simulink model "Test_21"  (R2024b)
settings: Solver=FixedStepAuto  StartTime=0.0  StopTime=50  RelTol=1e-3
undefined symbols (not defined in the file): BOOL, DINT, OTL, slplc
libraries: arduinolib x4
(part 2 of 10)

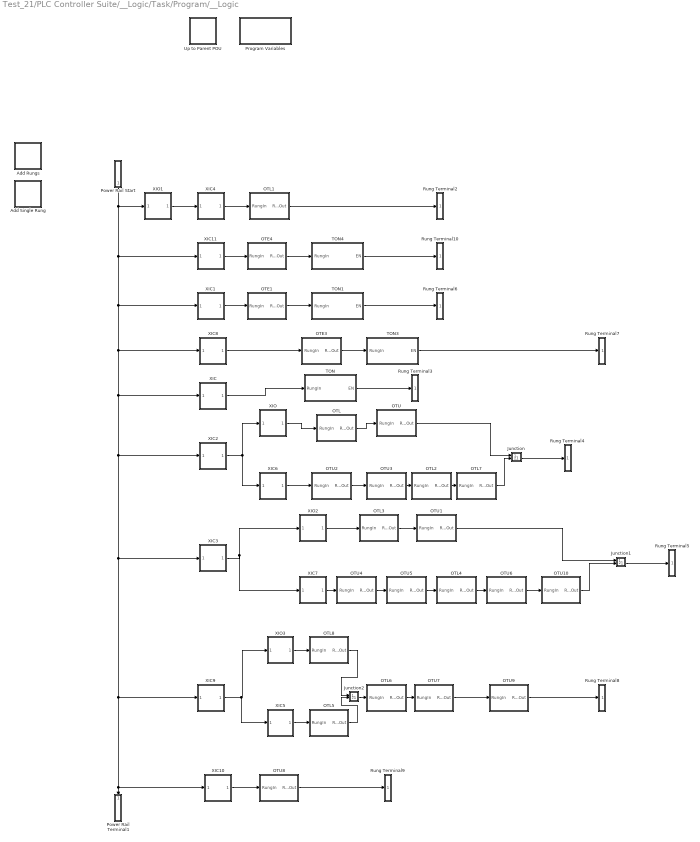
== system Test_21/PLC Controller Suite/__Logic/Task/Program/__Logic ==
  Add Rungs : Subsystem  DisableCoverage=on  TreatAsAtomicUnit=on  mask{PLCRungNumberToAdd=2, PLCBlockType=AddRungs}
      mask prompts: PLCRungNumberToAdd "Rung Number:"
      mask Help: web([docroot '/plccoder/ref/addrungs' '.html']);
      mask DialogControl PLCAddRungs Prompt: Add Rungs
      mask DialogControl PLCRungAddButton Prompt: Add
      mask DialogControl PLCRungAddButton Callback: slplc.callbacks.addLadderRungs(gcb);
      mask Display: disp(sprintf(['Add' newline 'Rungs']));
  Add Single Rung : Subsystem  DisableCoverage=on  TreatAsAtomicUnit=on  mask{PLCRungNumberToAdd=1, PLCBlockType=AddSingleRung}
      settings: OpenFcn=slplc.callbacks.addLadderRungs(gcb);
      mask Help: web([docroot '/plccoder/ref/addsinglerung' '.html']);
      mask DialogControl PLCAddRung Prompt: Add Single Rung
      mask Display: disp(sprintf(['Add' newline '1 Rung']));
  Junction : Subsystem  Priority=30  DisableCoverage=on  TreatAsAtomicUnit=on  mask{PLCBlockType=Junction, PLCPOUType=BranchJunction}
      mask Help: web([docroot '/plccoder/ref/junction' '.html']);
      mask DialogControl PLCBlockTitle Prompt: Rung Merge Point
      mask DialogControl PLCBlockDesc Prompt: This is the ladder diagram rung merge point.
  Junction1 : Subsystem  Priority=42  DisableCoverage=on  TreatAsAtomicUnit=on  mask{PLCBlockType=Junction, PLCPOUType=BranchJunction}
      mask Help: web([docroot '/plccoder/ref/junction' '.html']);
      mask DialogControl PLCBlockTitle Prompt: Rung Merge Point
      mask DialogControl PLCBlockDesc Prompt: This is the ladder diagram rung merge point.
  Junction2 : Subsystem  Priority=49  DisableCoverage=on  TreatAsAtomicUnit=on  mask{PLCBlockType=Junction, PLCPOUType=BranchJunction}
      mask Help: web([docroot '/plccoder/ref/junction' '.html']);
      mask DialogControl PLCBlockTitle Prompt: Rung Merge Point
      mask DialogControl PLCBlockDesc Prompt: This is the ladder diagram rung merge point.
  OTE1 : Subsystem  Priority=11  TreatAsAtomicUnit=on  mask{PLCOperandTag=Led2, PLCBlockType=OTE, PLCPOUType=Coil, PLCOperandExpression=xxx_PLC_VAR_Led2}
      mask prompts: PLCOperandTag "Operand Tag:"
      mask init:
      | slplc.callbacks.initInstruction(gcb);
      settings: AttributesFormatString=%<PLCOperandTag>
      mask Help: web([docroot '/plccoder/ref/ote' '.html']);
      mask DialogControl PLCBlockTitle Prompt: Output Energize (OTE)
  OTE3 : Subsystem  Priority=15  TreatAsAtomicUnit=on  mask{PLCOperandTag=Led3, PLCBlockType=OTE, PLCPOUType=Coil, PLCOperandExpression=xxx_PLC_VAR_Led3}
      mask prompts: PLCOperandTag "Operand Tag:"
      mask init:
      | slplc.callbacks.initInstruction(gcb);
      settings: AttributesFormatString=%<PLCOperandTag>
      mask Help: web([docroot '/plccoder/ref/ote' '.html']);
      mask DialogControl PLCBlockTitle Prompt: Output Energize (OTE)
  OTE4 : Subsystem  Priority=7  TreatAsAtomicUnit=on  mask{PLCOperandTag=Led1, PLCBlockType=OTE, PLCPOUType=Coil, PLCOperandExpression=xxx_PLC_VAR_Led1}
      mask prompts: PLCOperandTag "Operand Tag:"
      mask init:
      | slplc.callbacks.initInstruction(gcb);
      settings: AttributesFormatString=%<PLCOperandTag>
      mask Help: web([docroot '/plccoder/ref/ote' '.html']);
      mask DialogControl PLCBlockTitle Prompt: Output Energize (OTE)
  OTL : Subsystem  Priority=23  TreatAsAtomicUnit=on  mask{PLCOperandTag=B, PLCBlockType=OTL, PLCPOUType=Coil, PLCOperandExpression=xxx_PLC_VAR_B}
      mask prompts: PLCOperandTag "Operand Tag:"
      mask init:
      | slplc.callbacks.initInstruction(gcb);
      settings: AttributesFormatString=%<PLCOperandTag>
      mask Help: web([docroot '/plccoder/ref/otl' '.html']);
      mask DialogControl PLCBlockTitle Prompt: Output Latch (OTL)
      mask Display: disp('L');
  OTL1 : Subsystem  Priority=4  TreatAsAtomicUnit=on  mask{PLCOperandTag=ButtonLatch, PLCBlockType=OTL, PLCPOUType=Coil, PLCOperandExpression=xxx_PLC_VAR_ButtonLatch}
      mask prompts: PLCOperandTag "Operand Tag:"
      mask init:
      | slplc.callbacks.initInstruction(gcb);
      settings: AttributesFormatString=%<PLCOperandTag>
      mask Help: web([docroot '/plccoder/ref/otl' '.html']);
      mask DialogControl PLCBlockTitle Prompt: Output Latch (OTL)
      mask Display: disp('L');
  OTL2 : Subsystem  Priority=28  TreatAsAtomicUnit=on  mask{PLCOperandTag=C, PLCBlockType=OTL, PLCPOUType=Coil, PLCOperandExpression=xxx_PLC_VAR_C}
      mask prompts: PLCOperandTag "Operand Tag:"
      mask init:
      | slplc.callbacks.initInstruction(gcb);
      settings: AttributesFormatString=%<PLCOperandTag>
      mask Help: web([docroot '/plccoder/ref/otl' '.html']);
      mask DialogControl PLCBlockTitle Prompt: Output Latch (OTL)
      mask Display: disp('L');
  OTL3 : Subsystem  Priority=34  TreatAsAtomicUnit=on  mask{PLCOperandTag=A, PLCBlockType=OTL, PLCPOUType=Coil, PLCOperandExpression=xxx_PLC_VAR_A}
      mask prompts: PLCOperandTag "Operand Tag:"
      mask init:
      | slplc.callbacks.initInstruction(gcb);
      settings: AttributesFormatString=%<PLCOperandTag>
      mask Help: web([docroot '/plccoder/ref/otl' '.html']);
      mask DialogControl PLCBlockTitle Prompt: Output Latch (OTL)
      mask Display: disp('L');
  OTL4 : Subsystem  Priority=39  TreatAsAtomicUnit=on  mask{PLCOperandTag=C, PLCBlockType=OTL, PLCPOUType=Coil, PLCOperandExpression=xxx_PLC_VAR_C}
      mask prompts: PLCOperandTag "Operand Tag:"
      mask init:
      | slplc.callbacks.initInstruction(gcb);
      settings: AttributesFormatString=%<PLCOperandTag>
      mask Help: web([docroot '/plccoder/ref/otl' '.html']);
      mask DialogControl PLCBlockTitle Prompt: Output Latch (OTL)
      mask Display: disp('L');
  OTL5 : Subsystem  Priority=48  TreatAsAtomicUnit=on  mask{PLCOperandTag=B, PLCBlockType=OTL, PLCPOUType=Coil, PLCOperandExpression=xxx_PLC_VAR_B}
      mask prompts: PLCOperandTag "Operand Tag:"
      mask init:
      | slplc.callbacks.initInstruction(gcb);
      settings: AttributesFormatString=%<PLCOperandTag>
      mask Help: web([docroot '/plccoder/ref/otl' '.html']);
      mask DialogControl PLCBlockTitle Prompt: Output Latch (OTL)
      mask Display: disp('L');
  OTL6 : Subsystem  Priority=50  TreatAsAtomicUnit=on  mask{PLCOperandTag=BIgnore, PLCBlockType=OTL, PLCPOUType=Coil, PLCOperandExpression=xxx_PLC_VAR_BIgnore}
      mask prompts: PLCOperandTag "Operand Tag:"
      mask init:
      | slplc.callbacks.initInstruction(gcb);
      settings: AttributesFormatString=%<PLCOperandTag>
      mask Help: web([docroot '/plccoder/ref/otl' '.html']);
      mask DialogControl PLCBlockTitle Prompt: Output Latch (OTL)
      mask Display: disp('L');
  OTL7 : Subsystem  Priority=29  TreatAsAtomicUnit=on  mask{PLCOperandTag=StateLed1, PLCBlockType=OTL, PLCPOUType=Coil, PLCOperandExpression=xxx_PLC_VAR_StateLed1}
      mask prompts: PLCOperandTag "Operand Tag:"
      mask init:
      | slplc.callbacks.initInstruction(gcb);
      settings: AttributesFormatString=%<PLCOperandTag>
      mask Help: web([docroot '/plccoder/ref/otl' '.html']);
      mask DialogControl PLCBlockTitle Prompt: Output Latch (OTL)
      mask Display: disp('L');
  OTL8 : Subsystem  Priority=46  TreatAsAtomicUnit=on  mask{PLCOperandTag=A, PLCBlockType=OTL, PLCPOUType=Coil, PLCOperandExpression=xxx_PLC_VAR_A}
      mask prompts: PLCOperandTag "Operand Tag:"
      mask init:
      | slplc.callbacks.initInstruction(gcb);
      settings: AttributesFormatString=%<PLCOperandTag>
      mask Help: web([docroot '/plccoder/ref/otl' '.html']);
      mask DialogControl PLCBlockTitle Prompt: Output Latch (OTL)
      mask Display: disp('L');
  OTU : Subsystem  Priority=24  TreatAsAtomicUnit=on  mask{PLCOperandTag=A, PLCBlockType=OTU, PLCPOUType=Coil, PLCOperandExpression=xxx_PLC_VAR_A}
      mask prompts: PLCOperandTag "Operand Tag:"
      mask init:
      | slplc.callbacks.initInstruction(gcb);
      settings: AttributesFormatString=%<PLCOperandTag>
      mask Help: web([docroot '/plccoder/ref/otu' '.html']);
      mask DialogControl PLCBlockTitle Prompt: Output Unlatch (OTU)
      mask Display: disp('U');
  OTU1 : Subsystem  Priority=35  TreatAsAtomicUnit=on  mask{PLCOperandTag=B, PLCBlockType=OTU, PLCPOUType=Coil, PLCOperandExpression=xxx_PLC_VAR_B}
      mask prompts: PLCOperandTag "Operand Tag:"
      mask init:
      | slplc.callbacks.initInstruction(gcb);
      settings: AttributesFormatString=%<PLCOperandTag>
      mask Help: web([docroot '/plccoder/ref/otu' '.html']);
      mask DialogControl PLCBlockTitle Prompt: Output Unlatch (OTU)
      mask Display: disp('U');
  OTU10 : Subsystem  Priority=41  TreatAsAtomicUnit=on  mask{PLCOperandTag=StateLed1, PLCBlockType=OTU, PLCPOUType=Coil, PLCOperandExpression=xxx_PLC_VAR_StateLed1}
      mask prompts: PLCOperandTag "Operand Tag:"
      mask init:
      | slplc.callbacks.initInstruction(gcb);
      settings: AttributesFormatString=%<PLCOperandTag>
      mask Help: web([docroot '/plccoder/ref/otu' '.html']);
      mask DialogControl PLCBlockTitle Prompt: Output Unlatch (OTU)
      mask Display: disp('U');
  OTU2 : Subsystem  Priority=26  TreatAsAtomicUnit=on  mask{PLCOperandTag=A, PLCBlockType=OTU, PLCPOUType=Coil, PLCOperandExpression=xxx_PLC_VAR_A}
      mask prompts: PLCOperandTag "Operand Tag:"
      mask init:
      | slplc.callbacks.initInstruction(gcb);
      settings: AttributesFormatString=%<PLCOperandTag>
      mask Help: web([docroot '/plccoder/ref/otu' '.html']);
      mask DialogControl PLCBlockTitle Prompt: Output Unlatch (OTU)
      mask Display: disp('U');
  OTU3 : Subsystem  Priority=27  TreatAsAtomicUnit=on  mask{PLCOperandTag=B, PLCBlockType=OTU, PLCPOUType=Coil, PLCOperandExpression=xxx_PLC_VAR_B}
      mask prompts: PLCOperandTag "Operand Tag:"
      mask init:
      | slplc.callbacks.initInstruction(gcb);
      settings: AttributesFormatString=%<PLCOperandTag>
      mask Help: web([docroot '/plccoder/ref/otu' '.html']);
      mask DialogControl PLCBlockTitle Prompt: Output Unlatch (OTU)
      mask Display: disp('U');
  OTU4 : Subsystem  Priority=37  TreatAsAtomicUnit=on  mask{PLCOperandTag=A, PLCBlockType=OTU, PLCPOUType=Coil, PLCOperandExpression=xxx_PLC_VAR_A}
      mask prompts: PLCOperandTag "Operand Tag:"
      mask init:
      | slplc.callbacks.initInstruction(gcb);
      settings: AttributesFormatString=%<PLCOperandTag>
      mask Help: web([docroot '/plccoder/ref/otu' '.html']);
      mask DialogControl PLCBlockTitle Prompt: Output Unlatch (OTU)
      mask Display: disp('U');
  OTU5 : Subsystem  Priority=38  TreatAsAtomicUnit=on  mask{PLCOperandTag=B, PLCBlockType=OTU, PLCPOUType=Coil, PLCOperandExpression=xxx_PLC_VAR_B}
      mask prompts: PLCOperandTag "Operand Tag:"
      mask init:
      | slplc.callbacks.initInstruction(gcb);
      settings: AttributesFormatString=%<PLCOperandTag>
      mask Help: web([docroot '/plccoder/ref/otu' '.html']);
      mask DialogControl PLCBlockTitle Prompt: Output Unlatch (OTU)
      mask Display: disp('U');
  OTU6 : Subsystem  Priority=40  TreatAsAtomicUnit=on  mask{PLCOperandTag=ButtonLatch, PLCBlockType=OTU, PLCPOUType=Coil, PLCOperandExpression=xxx_PLC_VAR_ButtonLatch}
      mask prompts: PLCOperandTag "Operand Tag:"
      mask init:
      | slplc.callbacks.initInstruction(gcb);
      settings: AttributesFormatString=%<PLCOperandTag>
      mask Help: web([docroot '/plccoder/ref/otu' '.html']);
      mask DialogControl PLCBlockTitle Prompt: Output Unlatch (OTU)
      mask Display: disp('U');
  OTU7 : Subsystem  Priority=51  TreatAsAtomicUnit=on  mask{PLCOperandTag=ButtonLatch, PLCBlockType=OTU, PLCPOUType=Coil, PLCOperandExpression=xxx_PLC_VAR_ButtonLatch}
      mask prompts: PLCOperandTag "Operand Tag:"
      mask init:
      | slplc.callbacks.initInstruction(gcb);
      settings: AttributesFormatString=%<PLCOperandTag>
      mask Help: web([docroot '/plccoder/ref/otu' '.html']);
      mask DialogControl PLCBlockTitle Prompt: Output Unlatch (OTU)
      mask Display: disp('U');
  OTU8 : Subsystem  Priority=55  TreatAsAtomicUnit=on  mask{PLCOperandTag=BIgnore, PLCBlockType=OTU, PLCPOUType=Coil, PLCOperandExpression=xxx_PLC_VAR_BIgnore}
      mask prompts: PLCOperandTag "Operand Tag:"
      mask init:
      | slplc.callbacks.initInstruction(gcb);
      settings: AttributesFormatString=%<PLCOperandTag>
      mask Help: web([docroot '/plccoder/ref/otu' '.html']);
      mask DialogControl PLCBlockTitle Prompt: Output Unlatch (OTU)
      mask Display: disp('U');
  OTU9 : Subsystem  Priority=52  TreatAsAtomicUnit=on  mask{PLCOperandTag=C, PLCBlockType=OTU, PLCPOUType=Coil, PLCOperandExpression=xxx_PLC_VAR_C}
      mask prompts: PLCOperandTag "Operand Tag:"
      mask init:
      | slplc.callbacks.initInstruction(gcb);
      settings: AttributesFormatString=%<PLCOperandTag>
      mask Help: web([docroot '/plccoder/ref/otu' '.html']);
      mask DialogControl PLCBlockTitle Prompt: Output Unlatch (OTU)
      mask Display: disp('U');
  Power Rail Start : Subsystem  Priority=1  DisableCoverage=on  TreatAsAtomicUnit=on  mask{PLCBlockType=PowerRailStart}
      mask Help: web([docroot '/plccoder/ref/powerrailstart' '.html']);
      mask DialogControl PLCBlockTitle Prompt: Power Rail Start
      mask DialogControl PLCBlockDesc Prompt: This is the ladder diagram left power rail start block.
  Power Rail Terminal1 : Subsystem  DisableCoverage=on  TreatAsAtomicUnit=on  mask{PLCBlockType=PowerRailTerminal}
      mask Help: web([docroot '/plccoder/ref/powerrailterminal' '.html']);
      mask DialogControl PLCBlockTitle Prompt: Power Rail Terminal
      mask DialogControl PLCBlockDesc Prompt: This is the ladder diagram left power rail terminal block.
  Program Variables : Subsystem  Tag=ProgramVariableSS  DisableCoverage=on  TreatAsAtomicUnit=on  mask{PLCVarAName=A, PLCVarAScope=Local, PLCVarAPortType=Hidden, PLCVarAPortIndex=14, PLCVarADataType=BOOL, PLCVarASize=1, PLCVarAInitialValue=true, PLCVarAToDelete=off, PLCVarBName=B, PLCVarBScope=Local, PLCVarBPortType=Hidden, PLCVarBPortIndex=14, PLCVarBDataType=BOOL, PLCVarBSize=1, PLCVarBInitialValue=false, PLCVarBToDelete=off, PLCVarBIgnoreName=BIgnore, PLCVarBIgnoreScope=Local, PLCVarBIgnorePortType=Hidden, PLCVarBIgnorePortIndex=14, PLCVarBIgnoreDataType=BOOL, PLCVarBIgnoreSize=1, PLCVarBIgnoreInitialValue=false, PLCVarBIgnoreToDelete=off, PLCVarButtonLatchName=ButtonLatch, PLCVarButtonLatchScope=Local, PLCVarButtonLatchPortType=Hidden, PLCVarButtonLatchPortIndex=14, PLCVarButtonLatchDataType=BOOL, PLCVarButtonLatchSize=1, PLCVarButtonLatchInitialValue=false, PLCVarButtonLatchToDelete=off, PLCVarCName=C, PLCVarCScope=Local, PLCVarCPortType=Hidden, PLCVarCPortIndex=14, PLCVarCDataType=BOOL, PLCVarCSize=1, PLCVarCInitialValue=false, PLCVarCToDelete=off, PLCVarStateLed1Name=StateLed1, PLCVarStateLed1Scope=Local, PLCVarStateLed1PortType=Hidden, PLCVarStateLed1PortIndex=14, PLCVarStateLed1DataType=BOOL, PLCVarStateLed1Size=1, PLCVarStateLed1InitialValue=false, PLCVarStateLed1ToDelete=off, PLCVarT1Name=T1, PLCVarT1Scope=Local, PLCVarT1PortType=Hidden, PLCVarT1PortIndex=14, PLCVarT1DataType=Bus: TIMER, PLCVarT1Size=1, PLCVarT1InitialValue=T1_InitialValue, PLCVarT1ToDelete=off, PLCVarT2Name=T2, PLCVarT2Scope=Local, PLCVarT2PortType=Hidden, PLCVarT2PortIndex=14, PLCVarT2DataType=Bus: TIMER, PLCVarT2Size=1, PLCVarT2InitialValue=T1_InitialValue, PLCVarT2ToDelete=off, PLCVarT3Name=T3, PLCVarT3Scope=Local, PLCVarT3PortType=Hidden, PLCVarT3PortIndex=14, PLCVarT3DataType=Bus: TIMER, PLCVarT3Size=1, PLCVarT3InitialValue=T1_InitialValue, PLCVarT3ToDelete=off, PLCVarTBIgnoreName=TBIgnore, PLCVarTBIgnoreScope=Local, PLCVarTBIgnorePortType=Hidden, PLCVarTBIgnorePortIndex=14, PLCVarTBIgnoreDataType=Bus: TIMER, PLCVarTBIgnoreSize=1, PLCVarTBIgnoreInitialValue=T2_InitialValue, PLCVarTBIgnoreToDelete=off, PLCVarButtonName=Button, PLCVarButtonScope=External, PLCVarButtonPortType=Hidden, PLCVarButtonPortIndex=14, PLCVarButtonDataType=DINT, PLCVarButtonSize=-1, PLCVarButtonInitialValue=0, PLCVarButtonToDelete=off, PLCVarLed1Name=Led1, PLCVarLed1Scope=External, PLCVarLed1PortType=Hidden, PLCVarLed1PortIndex=14, PLCVarLed1DataType=DINT, PLCVarLed1Size=-1, PLCVarLed1InitialValue=0, PLCVarLed1ToDelete=off, PLCVarLed2Name=Led2, PLCVarLed2Scope=External, PLCVarLed2PortType=Hidden, PLCVarLed2PortIndex=14, PLCVarLed2DataType=DINT, PLCVarLed2Size=-1, PLCVarLed2InitialValue=0, PLCVarLed2ToDelete=off, PLCVarLed3Name=Led3, PLCVarLed3Scope=External, PLCVarLed3PortType=Hidden, PLCVarLed3PortIndex=14, PLCVarLed3DataType=DINT, PLCVarLed3Size=-1, PLCVarLed3InitialValue=0, PLCVarLed3ToDelete=off}
      mask init:
      | slplc.callbacks.initPOUVarSS(gcb);
      settings: OpenFcn=slplc.callbacks.openProgramVariableSS(gcb);
      mask Help: web([docroot '/plccoder/ref/programvariables' '.html']);
      mask TypeOptions PLCVarAScope: Local | External
      mask TypeOptions PLCVarAPortType: Hidden | Inport | Outport
      mask TypeOptions PLCVarAPortIndex: 1 | 2 | 3 | 4 | 5 | 6 | 7 | 8 | 9 | 10 | 11 | 12 | 13 | 14
      mask TypeOptions PLCVarBScope: Local | External
      mask TypeOptions PLCVarBPortType: Hidden | Inport | Outport
      mask TypeOptions PLCVarBPortIndex: 1 | 2 | 3 | 4 | 5 | 6 | 7 | 8 | 9 | 10 | 11 | 12 | 13 | 14
      mask TypeOptions PLCVarBIgnoreScope: Local | External
      mask TypeOptions PLCVarBIgnorePortType: Hidden | Inport | Outport
      mask TypeOptions PLCVarBIgnorePortIndex: 1 | 2 | 3 | 4 | 5 | 6 | 7 | 8 | 9 | 10 | 11 | 12 | 13 | 14
      mask TypeOptions PLCVarButtonLatchScope: Local | External
      mask TypeOptions PLCVarButtonLatchPortType: Hidden | Inport | Outport
      mask TypeOptions PLCVarButtonLatchPortIndex: 1 | 2 | 3 | 4 | 5 | 6 | 7 | 8 | 9 | 10 | 11 | 12 | 13 | 14
      mask TypeOptions PLCVarCScope: Local | External
      mask TypeOptions PLCVarCPortType: Hidden | Inport | Outport
      mask TypeOptions PLCVarCPortIndex: 1 | 2 | 3 | 4 | 5 | 6 | 7 | 8 | 9 | 10 | 11 | 12 | 13 | 14
      mask TypeOptions PLCVarStateLed1Scope: Local | External
      mask TypeOptions PLCVarStateLed1PortType: Hidden | Inport | Outport
      mask TypeOptions PLCVarStateLed1PortIndex: 1 | 2 | 3 | 4 | 5 | 6 | 7 | 8 | 9 | 10 | 11 | 12 | 13 | 14
      mask TypeOptions PLCVarT1Scope: Local | External
      mask TypeOptions PLCVarT1PortType: Hidden | Inport | Outport
      mask TypeOptions PLCVarT1PortIndex: 1 | 2 | 3 | 4 | 5 | 6 | 7 | 8 | 9 | 10 | 11 | 12 | 13 | 14
      mask TypeOptions PLCVarT2Scope: Local | External
      mask TypeOptions PLCVarT2PortType: Hidden | Inport | Outport
      mask TypeOptions PLCVarT2PortIndex: 1 | 2 | 3 | 4 | 5 | 6 | 7 | 8 | 9 | 10 | 11 | 12 | 13 | 14
      mask TypeOptions PLCVarT3Scope: Local | External
      mask TypeOptions PLCVarT3PortType: Hidden | Inport | Outport
      mask TypeOptions PLCVarT3PortIndex: 1 | 2 | 3 | 4 | 5 | 6 | 7 | 8 | 9 | 10 | 11 | 12 | 13 | 14
      mask TypeOptions PLCVarTBIgnoreScope: Local | External
      mask TypeOptions PLCVarTBIgnorePortType: Hidden | Inport | Outport
      mask TypeOptions PLCVarTBIgnorePortIndex: 1 | 2 | 3 | 4 | 5 | 6 | 7 | 8 | 9 | 10 | 11 | 12 | 13 | 14
      mask TypeOptions PLCVarButtonScope: Local | External
      mask TypeOptions PLCVarButtonPortType: Hidden | Inport | Outport
      mask TypeOptions PLCVarButtonPortIndex: 1 | 2 | 3 | 4 | 5 | 6 | 7 | 8 | 9 | 10 | 11 | 12 | 13 | 14
      mask TypeOptions PLCVarLed1Scope: Local | External
      mask TypeOptions PLCVarLed1PortType: Hidden | Inport | Outport
      mask TypeOptions PLCVarLed1PortIndex: 1 | 2 | 3 | 4 | 5 | 6 | 7 | 8 | 9 | 10 | 11 | 12 | 13 | 14
      mask TypeOptions PLCVarLed2Scope: Local | External
      mask TypeOptions PLCVarLed2PortType: Hidden | Inport | Outport
      mask TypeOptions PLCVarLed2PortIndex: 1 | 2 | 3 | 4 | 5 | 6 | 7 | 8 | 9 | 10 | 11 | 12 | 13 | 14
      mask TypeOptions PLCVarLed3Scope: Local | External
      mask TypeOptions PLCVarLed3PortType: Hidden | Inport | Outport
      mask TypeOptions PLCVarLed3PortIndex: 1 | 2 | 3 | 4 | 5 | 6 | 7 | 8 | 9 | 10 | 11 | 12 | 13 | 14
      mask DialogControl PLCBlockTitle Prompt: Program Variable Spreadsheet
      mask DialogControl PLCVarListHeaderName Prompt: Name
      mask DialogControl PLCVarListHeaderScope Prompt: Scope
      mask DialogControl PLCVarListHeaderDataType Prompt: Data Type
      mask DialogControl PLCVarListHeaderSize Prompt: Size
      mask DialogControl PLCVarListHeaderInitialValue Prompt: Initial Value
      mask DialogControl PLCVarListHeaderToDelete Prompt: Delete
  Rung Terminal10 : Subsystem  Priority=9  DisableCoverage=on  TreatAsAtomicUnit=on  mask{PLCRungTerminalIndex=2, PLCBlockType=RungTerminal}
      settings: AttributesFormatString=Rung %<PLCRungTerminalIndex>
      mask Help: web([docroot '/plccoder/ref/rungterminal' '.html']);
      mask DialogControl PLCBlockTitle Prompt: Rung Terminal
      mask DialogControl PLCBlockDescText Prompt: This is the ladder diagram rung terminal.
  Rung Terminal2 : Subsystem  Priority=5  DisableCoverage=on  TreatAsAtomicUnit=on  mask{PLCRungTerminalIndex=1, PLCBlockType=RungTerminal}
      settings: AttributesFormatString=Rung %<PLCRungTerminalIndex>
      mask Help: web([docroot '/plccoder/ref/rungterminal' '.html']);
      mask DialogControl PLCBlockTitle Prompt: Rung Terminal
      mask DialogControl PLCBlockDescText Prompt: This is the ladder diagram rung terminal.
  Rung Terminal3 : Subsystem  Priority=20  DisableCoverage=on  TreatAsAtomicUnit=on  mask{PLCRungTerminalIndex=5, PLCBlockType=RungTerminal}
      settings: AttributesFormatString=Rung %<PLCRungTerminalIndex>
      mask Help: web([docroot '/plccoder/ref/rungterminal' '.html']);
      mask DialogControl PLCBlockTitle Prompt: Rung Terminal
      mask DialogControl PLCBlockDescText Prompt: This is the ladder diagram rung terminal.
  Rung Terminal4 : Subsystem  Priority=31  DisableCoverage=on  TreatAsAtomicUnit=on  mask{PLCRungTerminalIndex=6, PLCBlockType=RungTerminal}
      settings: AttributesFormatString=Rung %<PLCRungTerminalIndex>
      mask Help: web([docroot '/plccoder/ref/rungterminal' '.html']);
      mask DialogControl PLCBlockTitle Prompt: Rung Terminal
      mask DialogControl PLCBlockDescText Prompt: This is the ladder diagram rung terminal.
  Rung Terminal5 : Subsystem  Priority=43  DisableCoverage=on  TreatAsAtomicUnit=on  mask{PLCRungTerminalIndex=7, PLCBlockType=RungTerminal}
      settings: AttributesFormatString=Rung %<PLCRungTerminalIndex>
      mask Help: web([docroot '/plccoder/ref/rungterminal' '.html']);
      mask DialogControl PLCBlockTitle Prompt: Rung Terminal
      mask DialogControl PLCBlockDescText Prompt: This is the ladder diagram rung terminal.
  Rung Terminal6 : Subsystem  Priority=13  DisableCoverage=on  TreatAsAtomicUnit=on  mask{PLCRungTerminalIndex=3, PLCBlockType=RungTerminal}
      settings: AttributesFormatString=Rung %<PLCRungTerminalIndex>
      mask Help: web([docroot '/plccoder/ref/rungterminal' '.html']);
      mask DialogControl PLCBlockTitle Prompt: Rung Terminal
      mask DialogControl PLCBlockDescText Prompt: This is the ladder diagram rung terminal.
  Rung Terminal7 : Subsystem  Priority=17  DisableCoverage=on  TreatAsAtomicUnit=on  mask{PLCRungTerminalIndex=4, PLCBlockType=RungTerminal}
      settings: AttributesFormatString=Rung %<PLCRungTerminalIndex>
      mask Help: web([docroot '/plccoder/ref/rungterminal' '.html']);
      mask DialogControl PLCBlockTitle Prompt: Rung Terminal
      mask DialogControl PLCBlockDescText Prompt: This is the ladder diagram rung terminal.
  Rung Terminal8 : Subsystem  Priority=53  DisableCoverage=on  TreatAsAtomicUnit=on  mask{PLCRungTerminalIndex=8, PLCBlockType=RungTerminal}
      settings: AttributesFormatString=Rung %<PLCRungTerminalIndex>
      mask Help: web([docroot '/plccoder/ref/rungterminal' '.html']);
      mask DialogControl PLCBlockTitle Prompt: Rung Terminal
      mask DialogControl PLCBlockDescText Prompt: This is the ladder diagram rung terminal.
  Rung Terminal9 : Subsystem  Priority=56  DisableCoverage=on  TreatAsAtomicUnit=on  mask{PLCRungTerminalIndex=9, PLCBlockType=RungTerminal}
      settings: AttributesFormatString=Rung %<PLCRungTerminalIndex>
      mask Help: web([docroot '/plccoder/ref/rungterminal' '.html']);
      mask DialogControl PLCBlockTitle Prompt: Rung Terminal
      mask DialogControl PLCBlockDescText Prompt: This is the ladder diagram rung terminal.
  TON : Subsystem  Priority=19  TreatAsAtomicUnit=on  mask{PLCOperandTag=TBIgnore, PLCTimerSampleTime=1, PLCBlockType=TON, PLCPOUType=stdFB, PLCOperandAccess=ReadWrite, PLCOperandExpression=xxx_PLC_VAR_TBIgnore}
      mask prompts: PLCOperandTag "Timer Tag:"; PLCTimerSampleTime "Timer Sample Time:"
      mask init:
      | block = gcb;
      | maskObj = Simulink.Mask.get(block);
      | maskObj.Display = sprintf('disp([''%s'' newline newline ''%s'']);', PLCBlockType, PLCOperandTag);
      | slplc.callbacks.initInstruction(block);
      settings: AttributesFormatString=%<PLCBlockType>: %<PLCOperandTag>
      mask Help: web([docroot '/plccoder/ref/ton' '.html']);
      mask DialogControl PLCBlockTitle Prompt: Timer On Delay (TON)
      mask Display: disp(['TON' newline newline 'TBIgnore']);
  TON1 : Subsystem  Priority=12  TreatAsAtomicUnit=on  mask{PLCOperandTag=T2, PLCTimerSampleTime=1, PLCBlockType=TON, PLCPOUType=stdFB, PLCOperandAccess=ReadWrite, PLCOperandExpression=xxx_PLC_VAR_T2}
      mask prompts: PLCOperandTag "Timer Tag:"; PLCTimerSampleTime "Timer Sample Time:"
      mask init:
      | block = gcb;
      | maskObj = Simulink.Mask.get(block);
      | maskObj.Display = sprintf('disp([''%s'' newline newline ''%s'']);', PLCBlockType, PLCOperandTag);
      | slplc.callbacks.initInstruction(block);
      settings: AttributesFormatString=%<PLCBlockType>: %<PLCOperandTag>
      mask Help: web([docroot '/plccoder/ref/ton' '.html']);
      mask DialogControl PLCBlockTitle Prompt: Timer On Delay (TON)
      mask Display: disp(['TON' newline newline 'T2']);
  TON3 : Subsystem  Priority=16  TreatAsAtomicUnit=on  mask{PLCOperandTag=T3, PLCTimerSampleTime=1, PLCBlockType=TON, PLCPOUType=stdFB, PLCOperandAccess=ReadWrite, PLCOperandExpression=xxx_PLC_VAR_T3}
      mask prompts: PLCOperandTag "Timer Tag:"; PLCTimerSampleTime "Timer Sample Time:"
      mask init:
      | block = gcb;
      | maskObj = Simulink.Mask.get(block);
      | maskObj.Display = sprintf('disp([''%s'' newline newline ''%s'']);', PLCBlockType, PLCOperandTag);
      | slplc.callbacks.initInstruction(block);
      settings: AttributesFormatString=%<PLCBlockType>: %<PLCOperandTag>
      mask Help: web([docroot '/plccoder/ref/ton' '.html']);
      mask DialogControl PLCBlockTitle Prompt: Timer On Delay (TON)
      mask Display: disp(['TON' newline newline 'T3']);
  TON4 : Subsystem  Priority=8  TreatAsAtomicUnit=on  mask{PLCOperandTag=T1, PLCTimerSampleTime=1, PLCBlockType=TON, PLCPOUType=stdFB, PLCOperandAccess=ReadWrite, PLCOperandExpression=xxx_PLC_VAR_T1}
      mask prompts: PLCOperandTag "Timer Tag:"; PLCTimerSampleTime "Timer Sample Time:"
      mask init:
      | block = gcb;
      | maskObj = Simulink.Mask.get(block);
      | maskObj.Display = sprintf('disp([''%s'' newline newline ''%s'']);', PLCBlockType, PLCOperandTag);
      | slplc.callbacks.initInstruction(block);
      settings: AttributesFormatString=%<PLCBlockType>: %<PLCOperandTag>
      mask Help: web([docroot '/plccoder/ref/ton' '.html']);
      mask DialogControl PLCBlockTitle Prompt: Timer On Delay (TON)
      mask Display: disp(['TON' newline newline 'T1']);
  Up to Parent POU : Subsystem  DisableCoverage=on  TreatAsAtomicUnit=on  mask{PLCBlockType=OpenParentPOU}
      settings: OpenFcn=slplc.callbacks.openParentPOUBlock(gcb);
      mask Help: web([docroot '/plccoder/ref/uptoparentpou' '.html']);
      mask DialogControl PLCBlockTitle Prompt: Add Single Rung
  XIC : Subsystem  Priority=18  TreatAsAtomicUnit=on  mask{PLCOperandTag=BIgnore, PLCBlockType=XIC, PLCPOUType=Contact, PLCOperandExpression=xxx_PLC_VAR_BIgnore}
      mask prompts: PLCOperandTag "Operand Tag:"
      mask init:
      | slplc.callbacks.initInstruction(gcb);
      settings: AttributesFormatString=%<PLCOperandTag>
      mask Help: web([docroot '/plccoder/ref/xic' '.html']);
      mask DialogControl PLCBlockTitle Prompt: Examine If Closed (XIC)
  XIC1 : Subsystem  Priority=10  TreatAsAtomicUnit=on  mask{PLCOperandTag=B, PLCBlockType=XIC, PLCPOUType=Contact, PLCOperandExpression=xxx_PLC_VAR_B}
      mask prompts: PLCOperandTag "Operand Tag:"
      mask init:
      | slplc.callbacks.initInstruction(gcb);
      settings: AttributesFormatString=%<PLCOperandTag>
      mask Help: web([docroot '/plccoder/ref/xic' '.html']);
      mask DialogControl PLCBlockTitle Prompt: Examine If Closed (XIC)
  XIC10 : Subsystem  Priority=54  TreatAsAtomicUnit=on  mask{PLCOperandTag=TBIgnore.DN, PLCBlockType=XIC, PLCPOUType=Contact, PLCOperandExpression=xxx_PLC_VAR_TBIgnore.DN}
      mask prompts: PLCOperandTag "Operand Tag:"
      mask init:
      | slplc.callbacks.initInstruction(gcb);
      settings: AttributesFormatString=%<PLCOperandTag>
      mask Help: web([docroot '/plccoder/ref/xic' '.html']);
      mask DialogControl PLCBlockTitle Prompt: Examine If Closed (XIC)
  XIC11 : Subsystem  Priority=6  TreatAsAtomicUnit=on  mask{PLCOperandTag=A, PLCBlockType=XIC, PLCPOUType=Contact, PLCOperandExpression=xxx_PLC_VAR_A}
      mask prompts: PLCOperandTag "Operand Tag:"
      mask init:
      | slplc.callbacks.initInstruction(gcb);
      settings: AttributesFormatString=%<PLCOperandTag>
      mask Help: web([docroot '/plccoder/ref/xic' '.html']);
      mask DialogControl PLCBlockTitle Prompt: Examine If Closed (XIC)
  XIC2 : Subsystem  Priority=21  TreatAsAtomicUnit=on  mask{PLCOperandTag=T1.DN, PLCBlockType=XIC, PLCPOUType=Contact, PLCOperandExpression=xxx_PLC_VAR_T1.DN}
      mask prompts: PLCOperandTag "Operand Tag:"
      mask init:
      | slplc.callbacks.initInstruction(gcb);
      settings: AttributesFormatString=%<PLCOperandTag>
      mask Help: web([docroot '/plccoder/ref/xic' '.html']);
      mask DialogControl PLCBlockTitle Prompt: Examine If Closed (XIC)
  XIC3 : Subsystem  Priority=32  TreatAsAtomicUnit=on  mask{PLCOperandTag=T2.DN, PLCBlockType=XIC, PLCPOUType=Contact, PLCOperandExpression=xxx_PLC_VAR_T2.DN}
      mask prompts: PLCOperandTag "Operand Tag:"
      mask init:
      | slplc.callbacks.initInstruction(gcb);
      settings: AttributesFormatString=%<PLCOperandTag>
      mask Help: web([docroot '/plccoder/ref/xic' '.html']);
      mask DialogControl PLCBlockTitle Prompt: Examine If Closed (XIC)
  XIC4 : Subsystem  Priority=3  TreatAsAtomicUnit=on  mask{PLCOperandTag=Button, PLCBlockType=XIC, PLCPOUType=Contact, PLCOperandExpression=xxx_PLC_VAR_Button}
      mask prompts: PLCOperandTag "Operand Tag:"
      mask init:
      | slplc.callbacks.initInstruction(gcb);
      settings: AttributesFormatString=%<PLCOperandTag>
      mask Help: web([docroot '/plccoder/ref/xic' '.html']);
      mask DialogControl PLCBlockTitle Prompt: Examine If Closed (XIC)
  XIC5 : Subsystem  Priority=47  TreatAsAtomicUnit=on  mask{PLCOperandTag=StateLed1, PLCBlockType=XIC, PLCPOUType=Contact, PLCOperandExpression=xxx_PLC_VAR_StateLed1}
      mask prompts: PLCOperandTag "Operand Tag:"
      mask init:
      | slplc.callbacks.initInstruction(gcb);
      settings: AttributesFormatString=%<PLCOperandTag>
      mask Help: web([docroot '/plccoder/ref/xic' '.html']);
      mask DialogControl PLCBlockTitle Prompt: Examine If Closed (XIC)
  XIC6 : Subsystem  Priority=25  TreatAsAtomicUnit=on  mask{PLCOperandTag=ButtonLatch, PLCBlockType=XIC, PLCPOUType=Contact, PLCOperandExpression=xxx_PLC_VAR_ButtonLatch}
      mask prompts: PLCOperandTag "Operand Tag:"
      mask init:
      | slplc.callbacks.initInstruction(gcb);
      settings: AttributesFormatString=%<PLCOperandTag>
      mask Help: web([docroot '/plccoder/ref/xic' '.html']);
      mask DialogControl PLCBlockTitle Prompt: Examine If Closed (XIC)
  XIC7 : Subsystem  Priority=36  TreatAsAtomicUnit=on  mask{PLCOperandTag=ButtonLatch, PLCBlockType=XIC, PLCPOUType=Contact, PLCOperandExpression=xxx_PLC_VAR_ButtonLatch}
      mask prompts: PLCOperandTag "Operand Tag:"
      mask init:
      | slplc.callbacks.initInstruction(gcb);
      settings: AttributesFormatString=%<PLCOperandTag>
      mask Help: web([docroot '/plccoder/ref/xic' '.html']);
      mask DialogControl PLCBlockTitle Prompt: Examine If Closed (XIC)
  XIC8 : Subsystem  Priority=14  TreatAsAtomicUnit=on  mask{PLCOperandTag=C, PLCBlockType=XIC, PLCPOUType=Contact, PLCOperandExpression=xxx_PLC_VAR_C}
      mask prompts: PLCOperandTag "Operand Tag:"
      mask init:
      | slplc.callbacks.initInstruction(gcb);
      settings: AttributesFormatString=%<PLCOperandTag>
      mask Help: web([docroot '/plccoder/ref/xic' '.html']);
      mask DialogControl PLCBlockTitle Prompt: Examine If Closed (XIC)
  XIC9 : Subsystem  Priority=44  TreatAsAtomicUnit=on  mask{PLCOperandTag=T3.DN, PLCBlockType=XIC, PLCPOUType=Contact, PLCOperandExpression=xxx_PLC_VAR_T3.DN}
      mask prompts: PLCOperandTag "Operand Tag:"
      mask init:
      | slplc.callbacks.initInstruction(gcb);
      settings: AttributesFormatString=%<PLCOperandTag>
      mask Help: web([docroot '/plccoder/ref/xic' '.html']);
      mask DialogControl PLCBlockTitle Prompt: Examine If Closed (XIC)
  XIO : Subsystem  Priority=22  TreatAsAtomicUnit=on  mask{PLCOperandExpression=xxx_PLC_VAR_ButtonLatch, PLCOperandTag=ButtonLatch, PLCBlockType=XIO, PLCPOUType=Contact}
      mask prompts: PLCOperandTag "Operand Tag:"
      mask init:
      | slplc.callbacks.initInstruction(gcb);
      settings: AttributesFormatString=%<PLCOperandTag>
      mask Help: web([docroot '/plccoder/ref/xio' '.html']);
      mask DialogControl PLCBlockTitle Prompt: Examine If Open (XIO)
  XIO1 : Subsystem  Priority=2  TreatAsAtomicUnit=on  mask{PLCOperandExpression=xxx_PLC_VAR_BIgnore, PLCOperandTag=BIgnore, PLCBlockType=XIO, PLCPOUType=Contact}
      mask prompts: PLCOperandTag "Operand Tag:"
      mask init:
      | slplc.callbacks.initInstruction(gcb);
      settings: AttributesFormatString=%<PLCOperandTag>
      mask Help: web([docroot '/plccoder/ref/xio' '.html']);
      mask DialogControl PLCBlockTitle Prompt: Examine If Open (XIO)
  XIO2 : Subsystem  Priority=33  TreatAsAtomicUnit=on  mask{PLCOperandExpression=xxx_PLC_VAR_ButtonLatch, PLCOperandTag=ButtonLatch, PLCBlockType=XIO, PLCPOUType=Contact}
      mask prompts: PLCOperandTag "Operand Tag:"
      mask init:
      | slplc.callbacks.initInstruction(gcb);
      settings: AttributesFormatString=%<PLCOperandTag>
      mask Help: web([docroot '/plccoder/ref/xio' '.html']);
      mask DialogControl PLCBlockTitle Prompt: Examine If Open (XIO)
  XIO3 : Subsystem  Priority=45  TreatAsAtomicUnit=on  mask{PLCOperandExpression=xxx_PLC_VAR_StateLed1, PLCOperandTag=StateLed1, PLCBlockType=XIO, PLCPOUType=Contact}
      mask prompts: PLCOperandTag "Operand Tag:"
      mask init:
      | slplc.callbacks.initInstruction(gcb);
      settings: AttributesFormatString=%<PLCOperandTag>
      mask Help: web([docroot '/plccoder/ref/xio' '.html']);
      mask DialogControl PLCBlockTitle Prompt: Examine If Open (XIO)
  wires:
  OTE4/1(RungOut) -> TON4/1(RungIn)
  XIC11/1(RungOut) -> OTE4/1(RungIn)
  OTE3/1(RungOut) -> TON3/1(RungIn)
  TON3/1(EN) -> Rung Terminal7/1(RungIn)
  XIC8/1(RungOut) -> OTE3/1(RungIn)
  XIC10/1(RungOut) -> OTU8/1(RungIn)
  XIO1/1(RungOut) -> XIC4/1(RungIn)
  XIC3/1(RungOut) -> XIO2/1(RungIn), XIC7/1(RungIn)
  XIC7/1(RungOut) -> OTU4/1(RungIn)
  OTU1/1(RungOut) -> Junction1/1(RungIn1)
  OTU/1(RungOut) -> Junction/1(RungIn1)
  OTU8/1(RungOut) -> Rung Terminal9/1(RungIn)
  XIC2/1(RungOut) -> XIO/1(RungIn), XIC6/1(RungIn)
  XIO/1(RungOut) -> OTL/1(RungIn)
  OTE1/1(RungOut) -> TON1/1(RungIn)
  OTU5/1(RungOut) -> OTL4/1(RungIn)
  XIC4/1(RungOut) -> OTL1/1(RungIn)
  OTU7/1(RungOut) -> OTU9/1(RungIn)
  OTU2/1(RungOut) -> OTU3/1(RungIn)
  Junction1/1(RungOut) -> Rung Terminal5/1(RungIn)
  OTL/1(RungOut) -> OTU/1(RungIn)
  OTU9/1(RungOut) -> Rung Terminal8/1(RungIn)
  OTL4/1(RungOut) -> OTU6/1(RungIn)
  Power Rail Start/1(PowerOut) -> XIO1/1(RungIn), XIC11/1(RungIn), XIC8/1(RungIn), XIC/1(RungIn), XIC9/1(RungIn), XIC10/1(RungIn), Power Rail Terminal1/1(PowerIn), XIC3/1(RungIn), XIC2/1(RungIn), XIC1/1(RungIn)
  TON/1(EN) -> Rung Terminal3/1(RungIn)
  Junction/1(RungOut) -> Rung Terminal4/1(RungIn)
  OTU6/1(RungOut) -> OTU10/1(RungIn)
  XIC/1(RungOut) -> TON/1(RungIn)
  OTL6/1(RungOut) -> OTU7/1(RungIn)
  XIC6/1(RungOut) -> OTU2/1(RungIn)
  OTL3/1(RungOut) -> OTU1/1(RungIn)
  TON1/1(EN) -> Rung Terminal6/1(RungIn)
  OTL1/1(RungOut) -> Rung Terminal2/1(RungIn)
  TON4/1(EN) -> Rung Terminal10/1(RungIn)
  XIO2/1(RungOut) -> OTL3/1(RungIn)
  XIC1/1(RungOut) -> OTE1/1(RungIn)
  OTU3/1(RungOut) -> OTL2/1(RungIn)
  OTU4/1(RungOut) -> OTU5/1(RungIn)
  OTL2/1(RungOut) -> OTL7/1(RungIn)
  OTL7/1(RungOut) -> Junction/2(RungIn2)
  OTU10/1(RungOut) -> Junction1/2(RungIn2)
  XIC9/1(RungOut) -> XIC5/1(RungIn), XIO3/1(RungIn)
  XIO3/1(RungOut) -> OTL8/1(RungIn)
  XIC5/1(RungOut) -> OTL5/1(RungIn)
  Junction2/1(RungOut) -> OTL6/1(RungIn)
  OTL8/1(RungOut) -> Junction2/1(RungIn1)
  OTL5/1(RungOut) -> Junction2/2(RungIn2)

== system Test_21/PLC Controller Suite/__Logic/Task/Program/__Logic/Add Rungs ==

== system Test_21/PLC Controller Suite/__Logic/Task/Program/__Logic/Add Single Rung ==

== system Test_21/PLC Controller Suite/__Logic/Task/Program/__Logic/Junction ==
  RungIn1 : Inport
  RungIn2 : Inport  Port=2
  BlockEnableRead : Subsystem  DisableCoverage=on  TreatAsAtomicUnit=on  mask{PLCLabelTag=_Block_Enable, PLCBlockType=BlockEnableRead}
      mask prompts: PLCLabelTag "Label Tag:"
      mask init:
      | block = gcb;
      | maskObj = Simulink.Mask.get(block);
      | maskObj.Display = sprintf('disp(''%s'');', PLCLabelTag);
      mask Help: web([docroot '/plccoder/ref/blockenableread' '.html']);
      mask DialogControl PLCBlockTitle Prompt: Block Enable Read
      mask Display: disp('_Block_Enable');
  __Enable : Subsystem  TreatAsAtomicUnit=on
  __Format : MATLAB Function  Tag=PLC_Format_Joint  Priority=20  DisableCoverage=on  InitFcn=slplc.utils.setBlockAppearance('reset', '', {'black', 'black'});  StopFcn=slplc.utils.setBlockAppearance('reset', '', {'black', 'black'});  TreatAsAtomicUnit=on
  RungOut : Outport  VectorParamsAs1DForOutWhenUnconnected=off
  wires:
  __Enable/1(RungOut) -> RungOut/1, __Format/2(RungOut)
  RungIn2/1 -> __Enable/2(RungIn2)
  RungIn1/1 -> __Enable/1(RungIn1)
  BlockEnableRead/1(Out1) -> __Enable/Enable, __Format/1(BlockEnable)

== system Test_21/PLC Controller Suite/__Logic/Task/Program/__Logic/Junction1 ==
  RungIn1 : Inport
  RungIn2 : Inport  Port=2
  BlockEnableRead : Subsystem  DisableCoverage=on  TreatAsAtomicUnit=on  mask{PLCLabelTag=_Block_Enable, PLCBlockType=BlockEnableRead}
      mask prompts: PLCLabelTag "Label Tag:"
      mask init:
      | block = gcb;
      | maskObj = Simulink.Mask.get(block);
      | maskObj.Display = sprintf('disp(''%s'');', PLCLabelTag);
      mask Help: web([docroot '/plccoder/ref/blockenableread' '.html']);
      mask DialogControl PLCBlockTitle Prompt: Block Enable Read
      mask Display: disp('_Block_Enable');
  __Enable : Subsystem  TreatAsAtomicUnit=on
  __Format : MATLAB Function  Tag=PLC_Format_Joint  Priority=20  DisableCoverage=on  InitFcn=slplc.utils.setBlockAppearance('reset', '', {'black', 'black'});  StopFcn=slplc.utils.setBlockAppearance('reset', '', {'black', 'black'});  TreatAsAtomicUnit=on
  RungOut : Outport  VectorParamsAs1DForOutWhenUnconnected=off
  wires:
  __Enable/1(RungOut) -> RungOut/1, __Format/2(RungOut)
  RungIn2/1 -> __Enable/2(RungIn2)
  RungIn1/1 -> __Enable/1(RungIn1)
  BlockEnableRead/1(Out1) -> __Enable/Enable, __Format/1(BlockEnable)

== system Test_21/PLC Controller Suite/__Logic/Task/Program/__Logic/Junction2 ==
  RungIn1 : Inport
  RungIn2 : Inport  Port=2
  BlockEnableRead : Subsystem  DisableCoverage=on  TreatAsAtomicUnit=on  mask{PLCLabelTag=_Block_Enable, PLCBlockType=BlockEnableRead}
      mask prompts: PLCLabelTag "Label Tag:"
      mask init:
      | block = gcb;
      | maskObj = Simulink.Mask.get(block);
      | maskObj.Display = sprintf('disp(''%s'');', PLCLabelTag);
      mask Help: web([docroot '/plccoder/ref/blockenableread' '.html']);
      mask DialogControl PLCBlockTitle Prompt: Block Enable Read
      mask Display: disp('_Block_Enable');
  __Enable : Subsystem  TreatAsAtomicUnit=on
  __Format : MATLAB Function  Tag=PLC_Format_Joint  Priority=20  DisableCoverage=on  InitFcn=slplc.utils.setBlockAppearance('reset', '', {'black', 'black'});  StopFcn=slplc.utils.setBlockAppearance('reset', '', {'black', 'black'});  TreatAsAtomicUnit=on
  RungOut : Outport  VectorParamsAs1DForOutWhenUnconnected=off
  wires:
  __Enable/1(RungOut) -> RungOut/1, __Format/2(RungOut)
  RungIn2/1 -> __Enable/2(RungIn2)
  RungIn1/1 -> __Enable/1(RungIn1)
  BlockEnableRead/1(Out1) -> __Enable/Enable, __Format/1(BlockEnable)

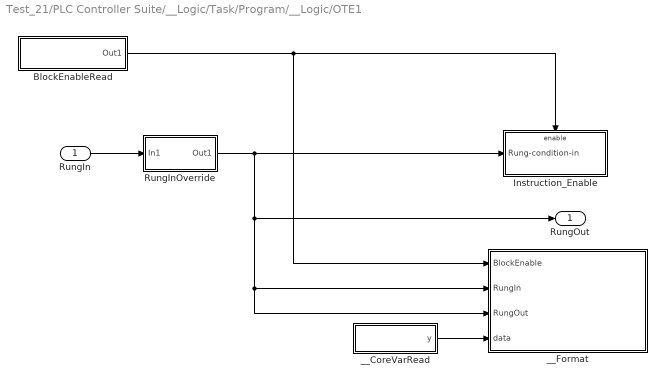
== system Test_21/PLC Controller Suite/__Logic/Task/Program/__Logic/OTE1 ==
  RungIn : Inport  PortDimensions=1
  BlockEnableRead : Subsystem  DisableCoverage=on  TreatAsAtomicUnit=on  mask{PLCLabelTag=_Block_Enable, PLCBlockType=BlockEnableRead}
      mask prompts: PLCLabelTag "Label Tag:"
      mask init:
      | block = gcb;
      | maskObj = Simulink.Mask.get(block);
      | maskObj.Display = sprintf('disp(''%s'');', PLCLabelTag);
      mask Help: web([docroot '/plccoder/ref/blockenableread' '.html']);
      mask DialogControl PLCBlockTitle Prompt: Block Enable Read
      mask Display: disp('_Block_Enable');
  Instruction_Enable : Subsystem  Priority=12  TreatAsAtomicUnit=on
  RungInOverride : Subsystem  DisableCoverage=on  TreatAsAtomicUnit=on
  __CoreVarRead : Subsystem  Tag=CoreVarReadBlock  DisableCoverage=on  TreatAsAtomicUnit=on  mask{PLCBlockType=CoreVarRead}
      mask init:
      | slplc.callbacks.initCoreVariable(gcb, 'read');
      mask Help: web([docroot '/plccoder/ref/__corevarread' '.html']);
      mask DialogControl PLCBlockTitle Prompt: Core Variable Read
  __Format : MATLAB Function  Tag=PLC_Format_Boolean  Priority=20  DisableCoverage=on  InitFcn=slplc.utils.setBlockAppearance('reset', '%<PLCOperandTag>');  StopFcn=slplc.utils.setBlockAppearance('reset', '%<PLCOperandTag>');  TreatAsAtomicUnit=on
  RungOut : Outport  OutDataTypeStr=BOOL  PortDimensions=1  InitialOutput=false  VectorParamsAs1DForOutWhenUnconnected=off
  wires:
  RungIn/1 -> RungInOverride/1(In1)
  BlockEnableRead/1(Out1) -> __Format/1(BlockEnable), Instruction_Enable/Enable
  RungInOverride/1(Out1) -> __Format/2(RungIn), __Format/3(RungOut), RungOut/1, Instruction_Enable/1(Rung-condition-in)
  __CoreVarRead/1(y) -> __Format/4(data)

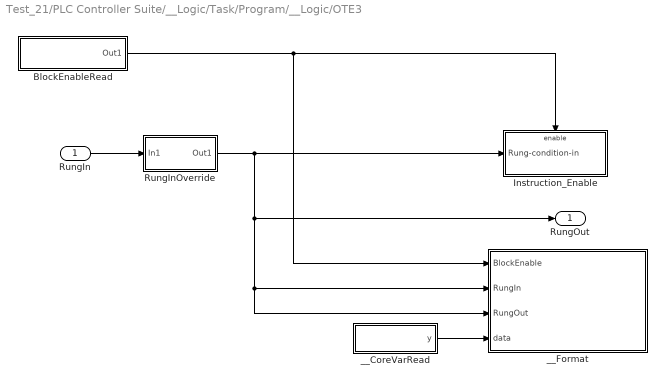
== system Test_21/PLC Controller Suite/__Logic/Task/Program/__Logic/OTE3 ==
  RungIn : Inport  PortDimensions=1
  BlockEnableRead : Subsystem  DisableCoverage=on  TreatAsAtomicUnit=on  mask{PLCLabelTag=_Block_Enable, PLCBlockType=BlockEnableRead}
      mask prompts: PLCLabelTag "Label Tag:"
      mask init:
      | block = gcb;
      | maskObj = Simulink.Mask.get(block);
      | maskObj.Display = sprintf('disp(''%s'');', PLCLabelTag);
      mask Help: web([docroot '/plccoder/ref/blockenableread' '.html']);
      mask DialogControl PLCBlockTitle Prompt: Block Enable Read
      mask Display: disp('_Block_Enable');
  Instruction_Enable : Subsystem  Priority=12  TreatAsAtomicUnit=on
  RungInOverride : Subsystem  DisableCoverage=on  TreatAsAtomicUnit=on
  __CoreVarRead : Subsystem  Tag=CoreVarReadBlock  DisableCoverage=on  TreatAsAtomicUnit=on  mask{PLCBlockType=CoreVarRead}
      mask init:
      | slplc.callbacks.initCoreVariable(gcb, 'read');
      mask Help: web([docroot '/plccoder/ref/__corevarread' '.html']);
      mask DialogControl PLCBlockTitle Prompt: Core Variable Read
  __Format : MATLAB Function  Tag=PLC_Format_Boolean  Priority=20  DisableCoverage=on  InitFcn=slplc.utils.setBlockAppearance('reset', '%<PLCOperandTag>');  StopFcn=slplc.utils.setBlockAppearance('reset', '%<PLCOperandTag>');  TreatAsAtomicUnit=on
  RungOut : Outport  OutDataTypeStr=BOOL  PortDimensions=1  InitialOutput=false  VectorParamsAs1DForOutWhenUnconnected=off
  wires:
  RungIn/1 -> RungInOverride/1(In1)
  BlockEnableRead/1(Out1) -> __Format/1(BlockEnable), Instruction_Enable/Enable
  RungInOverride/1(Out1) -> __Format/2(RungIn), __Format/3(RungOut), RungOut/1, Instruction_Enable/1(Rung-condition-in)
  __CoreVarRead/1(y) -> __Format/4(data)

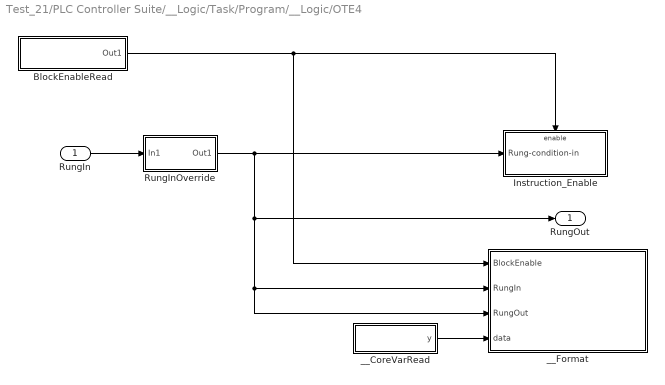
== system Test_21/PLC Controller Suite/__Logic/Task/Program/__Logic/OTE4 ==
  RungIn : Inport  PortDimensions=1
  BlockEnableRead : Subsystem  DisableCoverage=on  TreatAsAtomicUnit=on  mask{PLCLabelTag=_Block_Enable, PLCBlockType=BlockEnableRead}
      mask prompts: PLCLabelTag "Label Tag:"
      mask init:
      | block = gcb;
      | maskObj = Simulink.Mask.get(block);
      | maskObj.Display = sprintf('disp(''%s'');', PLCLabelTag);
      mask Help: web([docroot '/plccoder/ref/blockenableread' '.html']);
      mask DialogControl PLCBlockTitle Prompt: Block Enable Read
      mask Display: disp('_Block_Enable');
  Instruction_Enable : Subsystem  Priority=12  TreatAsAtomicUnit=on
  RungInOverride : Subsystem  DisableCoverage=on  TreatAsAtomicUnit=on
  __CoreVarRead : Subsystem  Tag=CoreVarReadBlock  DisableCoverage=on  TreatAsAtomicUnit=on  mask{PLCBlockType=CoreVarRead}
      mask init:
      | slplc.callbacks.initCoreVariable(gcb, 'read');
      mask Help: web([docroot '/plccoder/ref/__corevarread' '.html']);
      mask DialogControl PLCBlockTitle Prompt: Core Variable Read
  __Format : MATLAB Function  Tag=PLC_Format_Boolean  Priority=20  DisableCoverage=on  InitFcn=slplc.utils.setBlockAppearance('reset', '%<PLCOperandTag>');  StopFcn=slplc.utils.setBlockAppearance('reset', '%<PLCOperandTag>');  TreatAsAtomicUnit=on
  RungOut : Outport  OutDataTypeStr=BOOL  PortDimensions=1  InitialOutput=false  VectorParamsAs1DForOutWhenUnconnected=off
  wires:
  RungIn/1 -> RungInOverride/1(In1)
  BlockEnableRead/1(Out1) -> __Format/1(BlockEnable), Instruction_Enable/Enable
  RungInOverride/1(Out1) -> __Format/2(RungIn), __Format/3(RungOut), RungOut/1, Instruction_Enable/1(Rung-condition-in)
  __CoreVarRead/1(y) -> __Format/4(data)

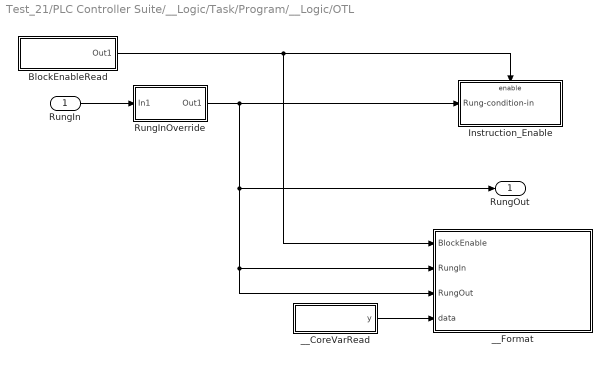
== system Test_21/PLC Controller Suite/__Logic/Task/Program/__Logic/OTL ==
  RungIn : Inport  PortDimensions=1
  BlockEnableRead : Subsystem  DisableCoverage=on  TreatAsAtomicUnit=on  mask{PLCLabelTag=_Block_Enable, PLCBlockType=BlockEnableRead}
      mask prompts: PLCLabelTag "Label Tag:"
      mask init:
      | block = gcb;
      | maskObj = Simulink.Mask.get(block);
      | maskObj.Display = sprintf('disp(''%s'');', PLCLabelTag);
      mask Help: web([docroot '/plccoder/ref/blockenableread' '.html']);
      mask DialogControl PLCBlockTitle Prompt: Block Enable Read
      mask Display: disp('_Block_Enable');
  Instruction_Enable : Subsystem  Priority=12  TreatAsAtomicUnit=on
  RungInOverride : Subsystem  DisableCoverage=on  TreatAsAtomicUnit=on
  __CoreVarRead : Subsystem  Tag=CoreVarReadBlock  DisableCoverage=on  TreatAsAtomicUnit=on  mask{PLCBlockType=CoreVarRead}
      mask init:
      | slplc.callbacks.initCoreVariable(gcb, 'read');
      mask Help: web([docroot '/plccoder/ref/__corevarread' '.html']);
      mask DialogControl PLCBlockTitle Prompt: Core Variable Read
  __Format : MATLAB Function  Tag=PLC_Format_Boolean  Priority=20  DisableCoverage=on  InitFcn=slplc.utils.setBlockAppearance('reset', '%<PLCOperandTag>');  StopFcn=slplc.utils.setBlockAppearance('reset', '%<PLCOperandTag>');  TreatAsAtomicUnit=on
  RungOut : Outport  OutDataTypeStr=BOOL  PortDimensions=1  InitialOutput=false  VectorParamsAs1DForOutWhenUnconnected=off
  wires:
  BlockEnableRead/1(Out1) -> Instruction_Enable/Enable, __Format/1(BlockEnable)
  RungIn/1 -> RungInOverride/1(In1)
  RungInOverride/1(Out1) -> Instruction_Enable/1(Rung-condition-in), __Format/3(RungOut), __Format/2(RungIn), RungOut/1
  __CoreVarRead/1(y) -> __Format/4(data)
